simulink model "dx_hand_model_rai3"  (R2017b)
settings: Solver=ode3  StartTime=0.0  StopTime=inf  FixedStep=0.01  RelTol=1e-3  EnableMultiTasking=on
InitFcn:
  | cutFreq = 0.1; % T
  | sampleTime = 0.01;
  | filt = tf(1,[cutFreq 1]);
  | filt = c2d(filt,sampleTime);
  | 
  | cutFreq2 = 1;
  | filt2 = tf(1,[cutFreq2 1]);
  | filt2 = c2d(filt2,sampleTime);
  | 
  | update_param = 2;
  | 
  | ampliFactor = 1.60;
  | ampliFactorMiddle = 2.00;
  | ampliFactorDistal = 1;
  | 
  | % Set Hand Address
  | RightHandAddress = '10.24.4.91';
  | Verosim = '10.100.39.22'
  | LeftHandAddress = '10.24.4.90'
  | 
  | max_force = 12; % Newton
model workspace (MAT data in the model file):
  SL_ROS_VariableLengthArrays_MaxSizes : struct (value not decoded)
libraries: robotlib x134, simulink_extras x28, simulink x16, dspnetwork x5, etargetslib x4
(part 10 of 19)

== matlab function dx_hand_model_rai3/Middle Finger/Jacobian Calculation/Middle Jacobian ==
  data: pose input; sensor input; measurements input; JTcomp output single; q_next output; q_pr input; J22_old input; J22_ol output
function [JTcomp, q_next, J22_ol] = fcn( pose, sensor, measurements, q_pr, J22_old)
% La funzione e' stata modificata da Antonio in data 6/06/2018
%
%#codegen
%
lx = sensor(1);
qB = sensor(2);

qo1 =pose(1);
qo2 =pose(2);
qK = pose(3);
qD = pose(4);
qG = pose(5);
qN = pose(6);
c1 = pose(7);
c2 = pose(8);

s_slitta = 13.5;

%POSE ESTIMATION VALUE
xL_mag = measurements(3); % Posizione lungo l'asse x di L rispetto a K [RIMISURA]
offset = measurements(4); % Distanza tra il giunto K e l'appoggio del metacarpo [RIMISURA]
LIIp = measurements(1); % Semispessore del metacarpo e della falange (da tarare)
LIIp = LIIp + s_slitta;
LJJp = LIIp; % semispessore della falangina (da tarare, non per forza uguale a LIIp)
LLM = measurements(2); % Lunghezza della falange
LAB =  measurements(5);
LBC =  measurements(6);
LCD =  measurements(7);
LDE =  measurements(8);
LEF =  measurements(9);
LBH =  measurements(10); 
LGH =  measurements(11);
LGF =  measurements(12);
LEJ =  measurements(13);
LCI =  measurements(14);
LKB =  measurements(15);
LKNy = measurements(16); %% MISURA
LKNx = measurements(17); %% MISURA
lact = measurements(18); %Lunghezza dell'attuatore. [RIMISURA]

% LIIp = 7;
% LJJp = LIIp;
% LLM = 50;
% offset = 3;
% xL = 10;

% f1 = LLM;
% f5 = xL;
% LBH = 37; 
% LKB = 35;
% LKH = LKB + LBH;
% LCI = 16;
% LGH =  86;
LHG =  LGH;
% LDE = 40;
% LAB =  18;   
% LEF =  27;
% LGF =  46;
% LCD =  9;
% LBC =  43;
% oy  = 134.8;
% ox  = 15; 
% LEJ =  39;
% off_fing = LIIp;  
% lact = 117.77;
% LKN =  135.6320;
% LNO = lact;
% LDF = LDE + LEF;
% LBD = LBC + LCD;


stepsize = 0.01;

%%NEWEST (Jacobian_StiffnessRenderingOptimization_Sim.mdl)
q_dif = (sensor - q_pr) / stepsize;
q_dif1 = q_dif(1);
q_dif2 = q_dif(2);


J11 = -(cos(qo1)*(LKB*cos(qK)+LBC*cos(qB-qK)-LCI*sin(qB-qK))-sin(qo1)*(LKB*sin(qK)-LBC*sin(qB-qK)-LCI*cos(qB-qK)))*((LDE+LEF)*sin(qo2)*cos(qB-qD-qG)*(LKB*sin(qK)-LBC*sin(qB-qK)-LCI*cos(qB-qK))+(LDE+LEF)*sin(qN)^2*cos(qB-qD-qG)*(cos(qo1)*sin(qo1+qo2)*(LKB*sin(qK)-LBC*sin(qB-qK))-LCI*cos(qo1)*sin(qo1+qo2)*cos(qB-qK)-sin(qo2)*(LKB*sin(qK)-LBC*sin(qB-qK)-LCI*cos(qB-qK))-sin(qo1)*cos(qo1+qo2)*(LKB*sin(qK)-LBC*sin(qB-qK)-LCI*cos(qB-qK)))-cos(qo1)*((LDE+LEF)*cos(qB-qD-qG)*(cos(qo1+qo2)*(LCD*cos(qB-qK)+LCI*sin(qB-qK)+LDE*cos(qB-qD-qK)-LEJ*sin(qB-qD-qK))-sin(qo1+qo2)*(LCI*cos(qB-qK)-LCD*sin(qB-qK)-LDE*sin(qB-qD-qK)-LEJ*cos(qB-qD-qK)))+(sin(qo1+qo2)*(LDE*sin(qB-qD-qK)+LEJ*cos(qB-qD-qK))+cos(qo1+qo2)*(LDE*cos(qB-qD-qK)-LEJ*sin(qB-qD-qK)))*(cos(qG-qK)*(LBH*cos(qK)+LHG*sin(qK)-LBC*cos(qB-qK)-LCD*cos(qB-qK)-LDE*cos(qB-qD-qK)-LEF*cos(qB-qD-qK))+sin(qG-qK)*(LHG*cos(qK)-LBH*sin(qK)-LBC*sin(qB-qK)-LCD*sin(qB-qK)-LDE*sin(qB-qD-qK)-LEF*sin(qB-qD-qK)))))/(cos(qN)*(LKB*sin(qK)+LAB*sin(qB-qK)-tan(qN)*(LKB*cos(qK)-LAB*cos(qB-qK)))*((LDE+LEF)*sin(qo1)*sin(qo2)*cos(qB-qD-qG)*(LIIp*cos(qo1)-c1*sin(qo1))*(LKB*sin(qK)-LBC*sin(qB-qK)-LCI*cos(qB-qK))-cos(qo1)*((LIIp*sin(qo1)+c1*cos(qo1))*((LDE+LEF)*sin(qo2)*cos(qB-qD-qG)*(LKB*sin(qK)-LBC*sin(qB-qK)-LCI*cos(qB-qK))-cos(qo1)*((LDE+LEF)*cos(qB-qD-qG)*(cos(qo1+qo2)*(LCD*cos(qB-qK)+LCI*sin(qB-qK)+LDE*cos(qB-qD-qK)-LEJ*sin(qB-qD-qK))-sin(qo1+qo2)*(LCI*cos(qB-qK)-LCD*sin(qB-qK)-LDE*sin(qB-qD-qK)-LEJ*cos(qB-qD-qK)))+(sin(qo1+qo2)*(LDE*sin(qB-qD-qK)+LEJ*cos(qB-qD-qK))+cos(qo1+qo2)*(LDE*cos(qB-qD-qK)-LEJ*sin(qB-qD-qK)))*(cos(qG-qK)*(LBH*cos(qK)+LHG*sin(qK)-LBC*cos(qB-qK)-LCD*cos(qB-qK)-LDE*cos(qB-qD-qK)-LEF*cos(qB-qD-qK))+sin(qG-qK)*(LHG*cos(qK)-LBH*sin(qK)-LBC*sin(qB-qK)-LCD*sin(qB-qK)-LDE*sin(qB-qD-qK)-LEF*sin(qB-qD-qK)))))-sin(qo1)*(LIIp*cos(qo1)-c1*sin(qo1))*((LDE+LEF)*sin(qo1+qo2)*cos(qB-qD-qG)*(LCI*cos(qB-qK)-LCD*sin(qB-qK)-LDE*sin(qB-qD-qK)-LEJ*cos(qB-qD-qK))-sin(qo1+qo2)*(LDE*sin(qB-qD-qK)+LEJ*cos(qB-qD-qK))*(cos(qG-qK)*(LBH*cos(qK)+LHG*sin(qK)-LBC*cos(qB-qK)-LCD*cos(qB-qK)-LDE*cos(qB-qD-qK)-LEF*cos(qB-qD-qK))+sin(qG-qK)*(LHG*cos(qK)-LBH*sin(qK)-LBC*sin(qB-qK)-LCD*sin(qB-qK)-LDE*sin(qB-qD-qK)-LEF*sin(qB-qD-qK)))-cos(qo1+qo2)*((LDE+LEF)*cos(qG-qK)*cos(qB-qD-qK)*(LCD*cos(qB-qK)+LCI*sin(qB-qK)+LDE*cos(qB-qD-qK)-LEJ*sin(qB-qD-qK))+cos(qG-qK)*(LDE*cos(qB-qD-qK)-LEJ*sin(qB-qD-qK))*(LBH*cos(qK)+LHG*sin(qK)-LBC*cos(qB-qK)-LCD*cos(qB-qK)-LDE*cos(qB-qD-qK)-LEF*cos(qB-qD-qK))+sin(qG-qK)*((LDE+LEF)*sin(qB-qD-qK)*(LCD*cos(qB-qK)+LCI*sin(qB-qK)+LDE*cos(qB-qD-qK)-LEJ*sin(qB-qD-qK))+(LDE*cos(qB-qD-qK)-LEJ*sin(qB-qD-qK))*(LHG*cos(qK)-LBH*sin(qK)-LBC*sin(qB-qK)-LCD*sin(qB-qK)-LDE*sin(qB-qD-qK)-LEF*sin(qB-qD-qK))))))));
J12 = cos(qo1)*((LDE+LEF)*sin(qo1+qo2)*cos(qB-qD-qG)*(LCI*cos(qB-qK)-LCD*sin(qB-qK)-LDE*sin(qB-qD-qK)-LEJ*cos(qB-qD-qK))*(cos(qo1)*(LKB*cos(qK)+LBC*cos(qB-qK)-LCI*sin(qB-qK))-sin(qo1)*(LKB*sin(qK)-LBC*sin(qB-qK)-LCI*cos(qB-qK)))+sin(qG-qK)*(LBC*sin(qB-qK)+LCD*sin(qB-qK)+LDE*sin(qB-qD-qK)+LEF*sin(qB-qD-qK))*(sin(qo1+qo2)*(LDE*sin(qB-qD-qK)+LEJ*cos(qB-qD-qK))+cos(qo1+qo2)*(LDE*cos(qB-qD-qK)-LEJ*sin(qB-qD-qK)))*(cos(qo1)*(LKB*cos(qK)+LBC*cos(qB-qK)-LCI*sin(qB-qK))-sin(qo1)*(LKB*sin(qK)-LBC*sin(qB-qK)-LCI*cos(qB-qK)))+cos(qG-qK)*(LBC*cos(qB-qK)+LCD*cos(qB-qK)+LDE*cos(qB-qD-qK)+LEF*cos(qB-qD-qK))*(sin(qo1+qo2)*(LDE*sin(qB-qD-qK)+LEJ*cos(qB-qD-qK))+cos(qo1+qo2)*(LDE*cos(qB-qD-qK)-LEJ*sin(qB-qD-qK)))*(cos(qo1)*(LKB*cos(qK)+LBC*cos(qB-qK)-LCI*sin(qB-qK))-sin(qo1)*(LKB*sin(qK)-LBC*sin(qB-qK)-LCI*cos(qB-qK)))-(LDE+LEF)*cos(qo1+qo2)*cos(qB-qD-qG)*(LCD*cos(qB-qK)+LCI*sin(qB-qK)+LDE*cos(qB-qD-qK)-LEJ*sin(qB-qD-qK))*(cos(qo1)*(LKB*cos(qK)+LBC*cos(qB-qK)-LCI*sin(qB-qK))-sin(qo1)*(LKB*sin(qK)-LBC*sin(qB-qK)-LCI*cos(qB-qK)))-(LBC*cos(qB-qK)-LCI*sin(qB-qK))*((LDE+LEF)*sin(qo2)*cos(qB-qD-qG)*(LKB*sin(qK)-LBC*sin(qB-qK)-LCI*cos(qB-qK))-cos(qo1)*((LDE+LEF)*cos(qB-qD-qG)*(cos(qo1+qo2)*(LCD*cos(qB-qK)+LCI*sin(qB-qK)+LDE*cos(qB-qD-qK)-LEJ*sin(qB-qD-qK))-sin(qo1+qo2)*(LCI*cos(qB-qK)-LCD*sin(qB-qK)-LDE*sin(qB-qD-qK)-LEJ*cos(qB-qD-qK)))+(sin(qo1+qo2)*(LDE*sin(qB-qD-qK)+LEJ*cos(qB-qD-qK))+cos(qo1+qo2)*(LDE*cos(qB-qD-qK)-LEJ*sin(qB-qD-qK)))*(cos(qG-qK)*(LBH*cos(qK)+LHG*sin(qK)-LBC*cos(qB-qK)-LCD*cos(qB-qK)-LDE*cos(qB-qD-qK)-LEF*cos(qB-qD-qK))+sin(qG-qK)*(LHG*cos(qK)-LBH*sin(qK)-LBC*sin(qB-qK)-LCD*sin(qB-qK)-LDE*sin(qB-qD-qK)-LEF*sin(qB-qD-qK)))))-(LBC*sin(qB-qK)+LCI*cos(qB-qK))*((LDE+LEF)*sin(qo2)*cos(qB-qD-qG)*(LKB*cos(qK)+LBC*cos(qB-qK)-LCI*sin(qB-qK))+sin(qo1)*((LDE+LEF)*sin(qo1+qo2)*cos(qB-qD-qG)*(LCI*cos(qB-qK)-LCD*sin(qB-qK)-LDE*sin(qB-qD-qK)-LEJ*cos(qB-qD-qK))-sin(qo1+qo2)*(LDE*sin(qB-qD-qK)+LEJ*cos(qB-qD-qK))*(cos(qG-qK)*(LBH*cos(qK)+LHG*sin(qK)-LBC*cos(qB-qK)-LCD*cos(qB-qK)-LDE*cos(qB-qD-qK)-LEF*cos(qB-qD-qK))+sin(qG-qK)*(LHG*cos(qK)-LBH*sin(qK)-LBC*sin(qB-qK)-LCD*sin(qB-qK)-LDE*sin(qB-qD-qK)-LEF*sin(qB-qD-qK)))-cos(qo1+qo2)*((LDE+LEF)*cos(qG-qK)*cos(qB-qD-qK)*(LCD*cos(qB-qK)+LCI*sin(qB-qK)+LDE*cos(qB-qD-qK)-LEJ*sin(qB-qD-qK))+cos(qG-qK)*(LDE*cos(qB-qD-qK)-LEJ*sin(qB-qD-qK))*(LBH*cos(qK)+LHG*sin(qK)-LBC*cos(qB-qK)-LCD*cos(qB-qK)-LDE*cos(qB-qD-qK)-LEF*cos(qB-qD-qK))+sin(qG-qK)*((LDE+LEF)*sin(qB-qD-qK)*(LCD*cos(qB-qK)+LCI*sin(qB-qK)+LDE*cos(qB-qD-qK)-LEJ*sin(qB-qD-qK))+(LDE*cos(qB-qD-qK)-LEJ*sin(qB-qD-qK))*(LHG*cos(qK)-LBH*sin(qK)-LBC*sin(qB-qK)-LCD*sin(qB-qK)-LDE*sin(qB-qD-qK)-LEF*sin(qB-qD-qK)))))))/((LDE+LEF)*sin(qo1)*sin(qo2)*cos(qB-qD-qG)*(LIIp*cos(qo1)-c1*sin(qo1))*(LKB*sin(qK)-LBC*sin(qB-qK)-LCI*cos(qB-qK))-cos(qo1)*((LIIp*sin(qo1)+c1*cos(qo1))*((LDE+LEF)*sin(qo2)*cos(qB-qD-qG)*(LKB*sin(qK)-LBC*sin(qB-qK)-LCI*cos(qB-qK))-cos(qo1)*((LDE+LEF)*cos(qB-qD-qG)*(cos(qo1+qo2)*(LCD*cos(qB-qK)+LCI*sin(qB-qK)+LDE*cos(qB-qD-qK)-LEJ*sin(qB-qD-qK))-sin(qo1+qo2)*(LCI*cos(qB-qK)-LCD*sin(qB-qK)-LDE*sin(qB-qD-qK)-LEJ*cos(qB-qD-qK)))+(sin(qo1+qo2)*(LDE*sin(qB-qD-qK)+LEJ*cos(qB-qD-qK))+cos(qo1+qo2)*(LDE*cos(qB-qD-qK)-LEJ*sin(qB-qD-qK)))*(cos(qG-qK)*(LBH*cos(qK)+LHG*sin(qK)-LBC*cos(qB-qK)-LCD*cos(qB-qK)-LDE*cos(qB-qD-qK)-LEF*cos(qB-qD-qK))+sin(qG-qK)*(LHG*cos(qK)-LBH*sin(qK)-LBC*sin(qB-qK)-LCD*sin(qB-qK)-LDE*sin(qB-qD-qK)-LEF*sin(qB-qD-qK)))))-sin(qo1)*(LIIp*cos(qo1)-c1*sin(qo1))*((LDE+LEF)*sin(qo1+qo2)*cos(qB-qD-qG)*(LCI*cos(qB-qK)-LCD*sin(qB-qK)-LDE*sin(qB-qD-qK)-LEJ*cos(qB-qD-qK))-sin(qo1+qo2)*(LDE*sin(qB-qD-qK)+LEJ*cos(qB-qD-qK))*(cos(qG-qK)*(LBH*cos(qK)+LHG*sin(qK)-LBC*cos(qB-qK)-LCD*cos(qB-qK)-LDE*cos(qB-qD-qK)-LEF*cos(qB-qD-qK))+sin(qG-qK)*(LHG*cos(qK)-LBH*sin(qK)-LBC*sin(qB-qK)-LCD*sin(qB-qK)-LDE*sin(qB-qD-qK)-LEF*sin(qB-qD-qK)))-cos(qo1+qo2)*((LDE+LEF)*cos(qG-qK)*cos(qB-qD-qK)*(LCD*cos(qB-qK)+LCI*sin(qB-qK)+LDE*cos(qB-qD-qK)-LEJ*sin(qB-qD-qK))+cos(qG-qK)*(LDE*cos(qB-qD-qK)-LEJ*sin(qB-qD-qK))*(LBH*cos(qK)+LHG*sin(qK)-LBC*cos(qB-qK)-LCD*cos(qB-qK)-LDE*cos(qB-qD-qK)-LEF*cos(qB-qD-qK))+sin(qG-qK)*((LDE+LEF)*sin(qB-qD-qK)*(LCD*cos(qB-qK)+LCI*sin(qB-qK)+LDE*cos(qB-qD-qK)-LEJ*sin(qB-qD-qK))+(LDE*cos(qB-qD-qK)-LEJ*sin(qB-qD-qK))*(LHG*cos(qK)-LBH*sin(qK)-LBC*sin(qB-qK)-LCD*sin(qB-qK)-LDE*sin(qB-qD-qK)-LEF*sin(qB-qD-qK))))))) - (cos(qo1)*(LKB*cos(qK)+LBC*cos(qB-qK)-LCI*sin(qB-qK))-sin(qo1)*(LKB*sin(qK)-LBC*sin(qB-qK)-LCI*cos(qB-qK)))*((LDE+LEF)*cos(qo1)*sin(qo1+qo2)*cos(qB-qD-qG)*(LKB*sin(qK)+LAB*sin(qB-qK)-tan(qN)*(LKB*cos(qK)-LAB*cos(qB-qK)))*(LCI*cos(qB-qK)-LCD*sin(qB-qK)-LDE*sin(qB-qD-qK)-LEJ*cos(qB-qD-qK))+cos(qo1)*sin(qG-qK)*(LKB*sin(qK)+LAB*sin(qB-qK)-tan(qN)*(LKB*cos(qK)-LAB*cos(qB-qK)))*(LBC*sin(qB-qK)+LCD*sin(qB-qK)+LDE*sin(qB-qD-qK)+LEF*sin(qB-qD-qK))*(sin(qo1+qo2)*(LDE*sin(qB-qD-qK)+LEJ*cos(qB-qD-qK))+cos(qo1+qo2)*(LDE*cos(qB-qD-qK)-LEJ*sin(qB-qD-qK)))+cos(qo1)*cos(qG-qK)*(LKB*sin(qK)+LAB*sin(qB-qK)-tan(qN)*(LKB*cos(qK)-LAB*cos(qB-qK)))*(LBC*cos(qB-qK)+LCD*cos(qB-qK)+LDE*cos(qB-qD-qK)+LEF*cos(qB-qD-qK))*(sin(qo1+qo2)*(LDE*sin(qB-qD-qK)+LEJ*cos(qB-qD-qK))+cos(qo1+qo2)*(LDE*cos(qB-qD-qK)-LEJ*sin(qB-qD-qK)))-(LDE+LEF)*sin(qo2)*cos(qB-qD-qG)*(LBC*sin(qB-qK)+LCI*cos(qB-qK))*(LKB*sin(qK)+LAB*sin(qB-qK)-tan(qN)*(LKB*cos(qK)-LAB*cos(qB-qK)))-(LDE+LEF)*cos(qo1)*cos(qo1+qo2)*cos(qB-qD-qG)*(LKB*sin(qK)+LAB*sin(qB-qK)-tan(qN)*(LKB*cos(qK)-LAB*cos(qB-qK)))*(LCD*cos(qB-qK)+LCI*sin(qB-qK)+LDE*cos(qB-qD-qK)-LEJ*sin(qB-qD-qK))-LAB*sin(qB-qK)*((LDE+LEF)*sin(qo2)*cos(qB-qD-qG)*(LKB*sin(qK)-LBC*sin(qB-qK)-LCI*cos(qB-qK))-cos(qo1)*((LDE+LEF)*cos(qB-qD-qG)*(cos(qo1+qo2)*(LCD*cos(qB-qK)+LCI*sin(qB-qK)+LDE*cos(qB-qD-qK)-LEJ*sin(qB-qD-qK))-sin(qo1+qo2)*(LCI*cos(qB-qK)-LCD*sin(qB-qK)-LDE*sin(qB-qD-qK)-LEJ*cos(qB-qD-qK)))+(sin(qo1+qo2)*(LDE*sin(qB-qD-qK)+LEJ*cos(qB-qD-qK))+cos(qo1+qo2)*(LDE*cos(qB-qD-qK)-LEJ*sin(qB-qD-qK)))*(cos(qG-qK)*(LBH*cos(qK)+LHG*sin(qK)-LBC*cos(qB-qK)-LCD*cos(qB-qK)-LDE*cos(qB-qD-qK)-LEF*cos(qB-qD-qK))+sin(qG-qK)*(LHG*cos(qK)-LBH*sin(qK)-LBC*sin(qB-qK)-LCD*sin(qB-qK)-LDE*sin(qB-qD-qK)-LEF*sin(qB-qD-qK)))))-LAB*tan(qN)*cos(qB-qK)*((LDE+LEF)*cos(qo1)*sin(qo1+qo2)*cos(qB-qD-qG)*(LKB*sin(qK)-LBC*sin(qB-qK)-LCD*sin(qB-qK)-LDE*sin(qB-qD-qK)-LEJ*cos(qB-qD-qK))-(LDE+LEF)*sin(qo1)*cos(qo1+qo2)*cos(qB-qD-qG)*(LKB*sin(qK)-LBC*sin(qB-qK)-LCI*cos(qB-qK))-cos(qo1)*sin(qo1+qo2)*(LDE*sin(qB-qD-qK)+LEJ*cos(qB-qD-qK))*(cos(qG-qK)*(LBH*cos(qK)+LHG*sin(qK)-LBC*cos(qB-qK)-LCD*cos(qB-qK)-LDE*cos(qB-qD-qK)-LEF*cos(qB-qD-qK))+sin(qG-qK)*(LHG*cos(qK)-LBH*sin(qK)-LBC*sin(qB-qK)-LCD*sin(qB-qK)-LDE*sin(qB-qD-qK)-LEF*sin(qB-qD-qK)))-cos(qo1)*cos(qo1+qo2)*((LDE+LEF)*cos(qG-qK)*cos(qB-qD-qK)*(LCD*cos(qB-qK)+LCI*sin(qB-qK)+LDE*cos(qB-qD-qK)-LEJ*sin(qB-qD-qK))+cos(qG-qK)*(LDE*cos(qB-qD-qK)-LEJ*sin(qB-qD-qK))*(LBH*cos(qK)+LHG*sin(qK)-LBC*cos(qB-qK)-LCD*cos(qB-qK)-LDE*cos(qB-qD-qK)-LEF*cos(qB-qD-qK))+sin(qG-qK)*((LDE+LEF)*sin(qB-qD-qK)*(LCD*cos(qB-qK)+LCI*sin(qB-qK)+LDE*cos(qB-qD-qK)-LEJ*sin(qB-qD-qK))+(LDE*cos(qB-qD-qK)-LEJ*sin(qB-qD-qK))*(LHG*cos(qK)-LBH*sin(qK)-LBC*sin(qB-qK)-LCD*sin(qB-qK)-LDE*sin(qB-qD-qK)-LEF*sin(qB-qD-qK))))))/((LKB*sin(qK)+LAB*sin(qB-qK)-tan(qN)*(LKB*cos(qK)-LAB*cos(qB-qK)))*((LDE+LEF)*sin(qo1)*sin(qo2)*cos(qB-qD-qG)*(LIIp*cos(qo1)-c1*sin(qo1))*(LKB*sin(qK)-LBC*sin(qB-qK)-LCI*cos(qB-qK))-cos(qo1)*((LIIp*sin(qo1)+c1*cos(qo1))*((LDE+LEF)*sin(qo2)*cos(qB-qD-qG)*(LKB*sin(qK)-LBC*sin(qB-qK)-LCI*cos(qB-qK))-cos(qo1)*((LDE+LEF)*cos(qB-qD-qG)*(cos(qo1+qo2)*(LCD*cos(qB-qK)+LCI*sin(qB-qK)+LDE*cos(qB-qD-qK)-LEJ*sin(qB-qD-qK))-sin(qo1+qo2)*(LCI*cos(qB-qK)-LCD*sin(qB-qK)-LDE*sin(qB-qD-qK)-LEJ*cos(qB-qD-qK)))+(sin(qo1+qo2)*(LDE*sin(qB-qD-qK)+LEJ*cos(qB-qD-qK))+cos(qo1+qo2)*(LDE*cos(qB-qD-qK)-LEJ*sin(qB-qD-qK)))*(cos(qG-qK)*(LBH*cos(qK)+LHG*sin(qK)-LBC*cos(qB-qK)-LCD*cos(qB-qK)-LDE*cos(qB-qD-qK)-LEF*cos(qB-qD-qK))+sin(qG-qK)*(LHG*cos(qK)-LBH*sin(qK)-LBC*sin(qB-qK)-LCD*sin(qB-qK)-LDE*sin(qB-qD-qK)-LEF*sin(qB-qD-qK)))))-sin(qo1)*(LIIp*cos(qo1)-c1*sin(qo1))*((LDE+LEF)*sin(qo1+qo2)*cos(qB-qD-qG)*(LCI*cos(qB-qK)-LCD*sin(qB-qK)-LDE*sin(qB-qD-qK)-LEJ*cos(qB-qD-qK))-sin(qo1+qo2)*(LDE*sin(qB-qD-qK)+LEJ*cos(qB-qD-qK))*(cos(qG-qK)*(LBH*cos(qK)+LHG*sin(qK)-LBC*cos(qB-qK)-LCD*cos(qB-qK)-LDE*cos(qB-qD-qK)-LEF*cos(qB-qD-qK))+sin(qG-qK)*(LHG*cos(qK)-LBH*sin(qK)-LBC*sin(qB-qK)-LCD*sin(qB-qK)-LDE*sin(qB-qD-qK)-LEF*sin(qB-qD-qK)))-cos(qo1+qo2)*((LDE+LEF)*cos(qG-qK)*cos(qB-qD-qK)*(LCD*cos(qB-qK)+LCI*sin(qB-qK)+LDE*cos(qB-qD-qK)-LEJ*sin(qB-qD-qK))+cos(qG-qK)*(LDE*cos(qB-qD-qK)-LEJ*sin(qB-qD-qK))*(LBH*cos(qK)+LHG*sin(qK)-LBC*cos(qB-qK)-LCD*cos(qB-qK)-LDE*cos(qB-qD-qK)-LEF*cos(qB-qD-qK))+sin(qG-qK)*((LDE+LEF)*sin(qB-qD-qK)*(LCD*cos(qB-qK)+LCI*sin(qB-qK)+LDE*cos(qB-qD-qK)-LEJ*sin(qB-qD-qK))+(LDE*cos(qB-qD-qK)-LEJ*sin(qB-qD-qK))*(LHG*cos(qK)-LBH*sin(qK)-LBC*sin(qB-qK)-LCD*sin(qB-qK)-LDE*sin(qB-qD-qK)-LEF*sin(qB-qD-qK))))))));
J21 = -(((LDE+LEF)*sin(qo2)*cos(qB-qD-qG)*(LKB*sin(qK)-LBC*sin(qB-qK)-LCI*cos(qB-qK))-cos(qo1)*((LDE+LEF)*cos(qB-qD-qG)*(cos(qo1+qo2)*(LCD*cos(qB-qK)+LCI*sin(qB-qK)+LDE*cos(qB-qD-qK)-LEJ*sin(qB-qD-qK))-sin(qo1+qo2)*(LCI*cos(qB-qK)-LCD*sin(qB-qK)-LDE*sin(qB-qD-qK)-LEJ*cos(qB-qD-qK)))+(sin(qo1+qo2)*(LDE*sin(qB-qD-qK)+LEJ*cos(qB-qD-qK))+cos(qo1+qo2)*(LDE*cos(qB-qD-qK)-LEJ*sin(qB-qD-qK)))*(cos(qG-qK)*(LBH*cos(qK)+LHG*sin(qK)-LBC*cos(qB-qK)-LCD*cos(qB-qK)-LDE*cos(qB-qD-qK)-LEF*cos(qB-qD-qK))+sin(qG-qK)*(LHG*cos(qK)-LBH*sin(qK)-LBC*sin(qB-qK)-LCD*sin(qB-qK)-LDE*sin(qB-qD-qK)-LEF*sin(qB-qD-qK)))))^2*(cos(qN)+sin(qN)^2*((LDE+LEF)*cos(qo1)*sin(qo1+qo2)*cos(qB-qD-qG)*(LKB*sin(qK)-LBC*sin(qB-qK)-LCD*sin(qB-qK)-LDE*sin(qB-qD-qK)-LEJ*cos(qB-qD-qK))-(LDE+LEF)*sin(qo1)*cos(qo1+qo2)*cos(qB-qD-qG)*(LKB*sin(qK)-LBC*sin(qB-qK)-LCI*cos(qB-qK))-cos(qo1)*sin(qo1+qo2)*(LDE*sin(qB-qD-qK)+LEJ*cos(qB-qD-qK))*(cos(qG-qK)*(LBH*cos(qK)+LHG*sin(qK)-LBC*cos(qB-qK)-LCD*cos(qB-qK)-LDE*cos(qB-qD-qK)-LEF*cos(qB-qD-qK))+sin(qG-qK)*(LHG*cos(qK)-LBH*sin(qK)-LBC*sin(qB-qK)-LCD*sin(qB-qK)-LDE*sin(qB-qD-qK)-LEF*sin(qB-qD-qK)))-cos(qo1)*cos(qo1+qo2)*((LDE+LEF)*cos(qG-qK)*cos(qB-qD-qK)*(LCD*cos(qB-qK)+LCI*sin(qB-qK)+LDE*cos(qB-qD-qK)-LEJ*sin(qB-qD-qK))+cos(qG-qK)*(LDE*cos(qB-qD-qK)-LEJ*sin(qB-qD-qK))*(LBH*cos(qK)+LHG*sin(qK)-LBC*cos(qB-qK)-LCD*cos(qB-qK)-LDE*cos(qB-qD-qK)-LEF*cos(qB-qD-qK))+sin(qG-qK)*((LDE+LEF)*sin(qB-qD-qK)*(LCD*cos(qB-qK)+LCI*sin(qB-qK)+LDE*cos(qB-qD-qK)-LEJ*sin(qB-qD-qK))+(LDE*cos(qB-qD-qK)-LEJ*sin(qB-qD-qK))*(LHG*cos(qK)-LBH*sin(qK)-LBC*sin(qB-qK)-LCD*sin(qB-qK)-LDE*sin(qB-qD-qK)-LEF*sin(qB-qD-qK)))))/(cos(qN)*((LDE+LEF)*sin(qo2)*cos(qB-qD-qG)*(LKB*sin(qK)-LBC*sin(qB-qK)-LCI*cos(qB-qK))-cos(qo1)*((LDE+LEF)*cos(qB-qD-qG)*(cos(qo1+qo2)*(LCD*cos(qB-qK)+LCI*sin(qB-qK)+LDE*cos(qB-qD-qK)-LEJ*sin(qB-qD-qK))-sin(qo1+qo2)*(LCI*cos(qB-qK)-LCD*sin(qB-qK)-LDE*sin(qB-qD-qK)-LEJ*cos(qB-qD-qK)))+(sin(qo1+qo2)*(LDE*sin(qB-qD-qK)+LEJ*cos(qB-qD-qK))+cos(qo1+qo2)*(LDE*cos(qB-qD-qK)-LEJ*sin(qB-qD-qK)))*(cos(qG-qK)*(LBH*cos(qK)+LHG*sin(qK)-LBC*cos(qB-qK)-LCD*cos(qB-qK)-LDE*cos(qB-qD-qK)-LEF*cos(qB-qD-qK))+sin(qG-qK)*(LHG*cos(qK)-LBH*sin(qK)-LBC*sin(qB-qK)-LCD*sin(qB-qK)-LDE*sin(qB-qD-qK)-LEF*sin(qB-qD-qK)))))))*(LIIp*sin(qo1)+c1*cos(qo1)+((LDE+LEF)*c2*cos(qB-qD-qG)*(cos(qo1)*(LKB*cos(qK)+LBC*cos(qB-qK)-LCI*sin(qB-qK))-sin(qo1)*(LKB*sin(qK)-LBC*sin(qB-qK)-LCI*cos(qB-qK)))+(LDE+LEF)*sin(qo1+qo2)*cos(qB-qD-qG)*(LIIp*cos(qo1)+sin(qo1)*(LLM-c1))*(cos(qo1)*(LKB*cos(qK)+LBC*cos(qB-qK)-LCI*sin(qB-qK))-sin(qo1)*(LKB*sin(qK)-LBC*sin(qB-qK)-LCI*cos(qB-qK)))-(LDE+LEF)*cos(qo1+qo2)*cos(qB-qD-qG)*(LIIp*sin(qo1)-cos(qo1)*(LLM-c1))*(cos(qo1)*(LKB*cos(qK)+LBC*cos(qB-qK)-LCI*sin(qB-qK))-sin(qo1)*(LKB*sin(qK)-LBC*sin(qB-qK)-LCI*cos(qB-qK)))-(LIIp*cos(qo1)-c1*sin(qo1))*((LDE+LEF)*sin(qo2)*cos(qB-qD-qG)*(LKB*cos(qK)+LBC*cos(qB-qK)-LCI*sin(qB-qK))+sin(qo1)*((LDE+LEF)*sin(qo1+qo2)*cos(qB-qD-qG)*(LCI*cos(qB-qK)-LCD*sin(qB-qK)-LDE*sin(qB-qD-qK)-LEJ*cos(qB-qD-qK))-sin(qo1+qo2)*(LDE*sin(qB-qD-qK)+LEJ*cos(qB-qD-qK))*(cos(qG-qK)*(LBH*cos(qK)+LHG*sin(qK)-LBC*cos(qB-qK)-LCD*cos(qB-qK)-LDE*cos(qB-qD-qK)-LEF*cos(qB-qD-qK))+sin(qG-qK)*(LHG*cos(qK)-LBH*sin(qK)-LBC*sin(qB-qK)-LCD*sin(qB-qK)-LDE*sin(qB-qD-qK)-LEF*sin(qB-qD-qK)))-cos(qo1+qo2)*((LDE+LEF)*cos(qG-qK)*cos(qB-qD-qK)*(LCD*cos(qB-qK)+LCI*sin(qB-qK)+LDE*cos(qB-qD-qK)-LEJ*sin(qB-qD-qK))+cos(qG-qK)*(LDE*cos(qB-qD-qK)-LEJ*sin(qB-qD-qK))*(LBH*cos(qK)+LHG*sin(qK)-LBC*cos(qB-qK)-LCD*cos(qB-qK)-LDE*cos(qB-qD-qK)-LEF*cos(qB-qD-qK))+sin(qG-qK)*((LDE+LEF)*sin(qB-qD-qK)*(LCD*cos(qB-qK)+LCI*sin(qB-qK)+LDE*cos(qB-qD-qK)-LEJ*sin(qB-qD-qK))+(LDE*cos(qB-qD-qK)-LEJ*sin(qB-qD-qK))*(LHG*cos(qK)-LBH*sin(qK)-LBC*sin(qB-qK)-LCD*sin(qB-qK)-LDE*sin(qB-qD-qK)-LEF*sin(qB-qD-qK)))))))/((LDE+LEF)*sin(qo2)*cos(qB-qD-qG)*(LKB*sin(qK)-LBC*sin(qB-qK)-LCI*cos(qB-qK))-cos(qo1)*((LDE+LEF)*cos(qB-qD-qG)*(cos(qo1+qo2)*(LCD*cos(qB-qK)+LCI*sin(qB-qK)+LDE*cos(qB-qD-qK)-LEJ*sin(qB-qD-qK))-sin(qo1+qo2)*(LCI*cos(qB-qK)-LCD*sin(qB-qK)-LDE*sin(qB-qD-qK)-LEJ*cos(qB-qD-qK)))+(sin(qo1+qo2)*(LDE*sin(qB-qD-qK)+LEJ*cos(qB-qD-qK))+cos(qo1+qo2)*(LDE*cos(qB-qD-qK)-LEJ*sin(qB-qD-qK)))*(cos(qG-qK)*(LBH*cos(qK)+LHG*sin(qK)-LBC*cos(qB-qK)-LCD*cos(qB-qK)-LDE*cos(qB-qD-qK)-LEF*cos(qB-qD-qK))+sin(qG-qK)*(LHG*cos(qK)-LBH*sin(qK)-LBC*sin(qB-qK)-LCD*sin(qB-qK)-LDE*sin(qB-qD-qK)-LEF*sin(qB-qD-qK))))))/((LDE+LEF)*c2*cos(qB-qD-qG)*(LKB*sin(qK)+LAB*sin(qB-qK)-tan(qN)*(LKB*cos(qK)-LAB*cos(qB-qK)))*((LDE+LEF)*sin(qo1)*sin(qo2)*cos(qB-qD-qG)*(LIIp*cos(qo1)-c1*sin(qo1))*(LKB*sin(qK)-LBC*sin(qB-qK)-LCI*cos(qB-qK))-cos(qo1)*((LIIp*sin(qo1)+c1*cos(qo1))*((LDE+LEF)*sin(qo2)*cos(qB-qD-qG)*(LKB*sin(qK)-LBC*sin(qB-qK)-LCI*cos(qB-qK))-cos(qo1)*((LDE+LEF)*cos(qB-qD-qG)*(cos(qo1+qo2)*(LCD*cos(qB-qK)+LCI*sin(qB-qK)+LDE*cos(qB-qD-qK)-LEJ*sin(qB-qD-qK))-sin(qo1+qo2)*(LCI*cos(qB-qK)-LCD*sin(qB-qK)-LDE*sin(qB-qD-qK)-LEJ*cos(qB-qD-qK)))+(sin(qo1+qo2)*(LDE*sin(qB-qD-qK)+LEJ*cos(qB-qD-qK))+cos(qo1+qo2)*(LDE*cos(qB-qD-qK)-LEJ*sin(qB-qD-qK)))*(cos(qG-qK)*(LBH*cos(qK)+LHG*sin(qK)-LBC*cos(qB-qK)-LCD*cos(qB-qK)-LDE*cos(qB-qD-qK)-LEF*cos(qB-qD-qK))+sin(qG-qK)*(LHG*cos(qK)-LBH*sin(qK)-LBC*sin(qB-qK)-LCD*sin(qB-qK)-LDE*sin(qB-qD-qK)-LEF*sin(qB-qD-qK)))))-sin(qo1)*(LIIp*cos(qo1)-c1*sin(qo1))*((LDE+LEF)*sin(qo1+qo2)*cos(qB-qD-qG)*(LCI*cos(qB-qK)-LCD*sin(qB-qK)-LDE*sin(qB-qD-qK)-LEJ*cos(qB-qD-qK))-sin(qo1+qo2)*(LDE*sin(qB-qD-qK)+LEJ*cos(qB-qD-qK))*(cos(qG-qK)*(LBH*cos(qK)+LHG*sin(qK)-LBC*cos(qB-qK)-LCD*cos(qB-qK)-LDE*cos(qB-qD-qK)-LEF*cos(qB-qD-qK))+sin(qG-qK)*(LHG*cos(qK)-LBH*sin(qK)-LBC*sin(qB-qK)-LCD*sin(qB-qK)-LDE*sin(qB-qD-qK)-LEF*sin(qB-qD-qK)))-cos(qo1+qo2)*((LDE+LEF)*cos(qG-qK)*cos(qB-qD-qK)*(LCD*cos(qB-qK)+LCI*sin(qB-qK)+LDE*cos(qB-qD-qK)-LEJ*sin(qB-qD-qK))+cos(qG-qK)*(LDE*cos(qB-qD-qK)-LEJ*sin(qB-qD-qK))*(LBH*cos(qK)+LHG*sin(qK)-LBC*cos(qB-qK)-LCD*cos(qB-qK)-LDE*cos(qB-qD-qK)-LEF*cos(qB-qD-qK))+sin(qG-qK)*((LDE+LEF)*sin(qB-qD-qK)*(LCD*cos(qB-qK)+LCI*sin(qB-qK)+LDE*cos(qB-qD-qK)-LEJ*sin(qB-qD-qK))+(LDE*cos(qB-qD-qK)-LEJ*sin(qB-qD-qK))*(LHG*cos(qK)-LBH*sin(qK)-LBC*sin(qB-qK)-LCD*sin(qB-qK)-LDE*sin(qB-qD-qK)-LEF*sin(qB-qD-qK)))))))));
J22_c = (-(c2*cos(qo1)+cos(qo1)*sin(qo1+qo2)*(LIIp*cos(qo1)+sin(qo1)*(LLM-c1))-sin(qo2)*(LIIp*cos(qo1)-c1*sin(qo1))-cos(qo1)*cos(qo1+qo2)*(LIIp*sin(qo1)-cos(qo1)*(LLM-c1)))*((LDE+LEF)*sin(qo1+qo2)*cos(qB-qD-qG)*(LCI*cos(qB-qK)-LCD*sin(qB-qK)-LDE*sin(qB-qD-qK)-LEJ*cos(qB-qD-qK))*(cos(qo1)*(LKB*cos(qK)+LBC*cos(qB-qK)-LCI*sin(qB-qK))-sin(qo1)*(LKB*sin(qK)-LBC*sin(qB-qK)-LCI*cos(qB-qK)))+sin(qG-qK)*(LBC*sin(qB-qK)+LCD*sin(qB-qK)+LDE*sin(qB-qD-qK)+LEF*sin(qB-qD-qK))*(sin(qo1+qo2)*(LDE*sin(qB-qD-qK)+LEJ*cos(qB-qD-qK))+cos(qo1+qo2)*(LDE*cos(qB-qD-qK)-LEJ*sin(qB-qD-qK)))*(cos(qo1)*(LKB*cos(qK)+LBC*cos(qB-qK)-LCI*sin(qB-qK))-sin(qo1)*(LKB*sin(qK)-LBC*sin(qB-qK)-LCI*cos(qB-qK)))+cos(qG-qK)*(LBC*cos(qB-qK)+LCD*cos(qB-qK)+LDE*cos(qB-qD-qK)+LEF*cos(qB-qD-qK))*(sin(qo1+qo2)*(LDE*sin(qB-qD-qK)+LEJ*cos(qB-qD-qK))+cos(qo1+qo2)*(LDE*cos(qB-qD-qK)-LEJ*sin(qB-qD-qK)))*(cos(qo1)*(LKB*cos(qK)+LBC*cos(qB-qK)-LCI*sin(qB-qK))-sin(qo1)*(LKB*sin(qK)-LBC*sin(qB-qK)-LCI*cos(qB-qK)))-(LDE+LEF)*cos(qo1+qo2)*cos(qB-qD-qG)*(LCD*cos(qB-qK)+LCI*sin(qB-qK)+LDE*cos(qB-qD-qK)-LEJ*sin(qB-qD-qK))*(cos(qo1)*(LKB*cos(qK)+LBC*cos(qB-qK)-LCI*sin(qB-qK))-sin(qo1)*(LKB*sin(qK)-LBC*sin(qB-qK)-LCI*cos(qB-qK)))-(LBC*cos(qB-qK)-LCI*sin(qB-qK))*((LDE+LEF)*sin(qo2)*cos(qB-qD-qG)*(LKB*sin(qK)-LBC*sin(qB-qK)-LCI*cos(qB-qK))-cos(qo1)*((LDE+LEF)*cos(qB-qD-qG)*(cos(qo1+qo2)*(LCD*cos(qB-qK)+LCI*sin(qB-qK)+LDE*cos(qB-qD-qK)-LEJ*sin(qB-qD-qK))-sin(qo1+qo2)*(LCI*cos(qB-qK)-LCD*sin(qB-qK)-LDE*sin(qB-qD-qK)-LEJ*cos(qB-qD-qK)))+(sin(qo1+qo2)*(LDE*sin(qB-qD-qK)+LEJ*cos(qB-qD-qK))+cos(qo1+qo2)*(LDE*cos(qB-qD-qK)-LEJ*sin(qB-qD-qK)))*(cos(qG-qK)*(LBH*cos(qK)+LHG*sin(qK)-LBC*cos(qB-qK)-LCD*cos(qB-qK)-LDE*cos(qB-qD-qK)-LEF*cos(qB-qD-qK))+sin(qG-qK)*(LHG*cos(qK)-LBH*sin(qK)-LBC*sin(qB-qK)-LCD*sin(qB-qK)-LDE*sin(qB-qD-qK)-LEF*sin(qB-qD-qK)))))-(LBC*sin(qB-qK)+LCI*cos(qB-qK))*((LDE+LEF)*sin(qo2)*cos(qB-qD-qG)*(LKB*cos(qK)+LBC*cos(qB-qK)-LCI*sin(qB-qK))+sin(qo1)*((LDE+LEF)*sin(qo1+qo2)*cos(qB-qD-qG)*(LCI*cos(qB-qK)-LCD*sin(qB-qK)-LDE*sin(qB-qD-qK)-LEJ*cos(qB-qD-qK))-sin(qo1+qo2)*(LDE*sin(qB-qD-qK)+LEJ*cos(qB-qD-qK))*(cos(qG-qK)*(LBH*cos(qK)+LHG*sin(qK)-LBC*cos(qB-qK)-LCD*cos(qB-qK)-LDE*cos(qB-qD-qK)-LEF*cos(qB-qD-qK))+sin(qG-qK)*(LHG*cos(qK)-LBH*sin(qK)-LBC*sin(qB-qK)-LCD*sin(qB-qK)-LDE*sin(qB-qD-qK)-LEF*sin(qB-qD-qK)))-cos(qo1+qo2)*((LDE+LEF)*cos(qG-qK)*cos(qB-qD-qK)*(LCD*cos(qB-qK)+LCI*sin(qB-qK)+LDE*cos(qB-qD-qK)-LEJ*sin(qB-qD-qK))+cos(qG-qK)*(LDE*cos(qB-qD-qK)-LEJ*sin(qB-qD-qK))*(LBH*cos(qK)+LHG*sin(qK)-LBC*cos(qB-qK)-LCD*cos(qB-qK)-LDE*cos(qB-qD-qK)-LEF*cos(qB-qD-qK))+sin(qG-qK)*((LDE+LEF)*sin(qB-qD-qK)*(LCD*cos(qB-qK)+LCI*sin(qB-qK)+LDE*cos(qB-qD-qK)-LEJ*sin(qB-qD-qK))+(LDE*cos(qB-qD-qK)-LEJ*sin(qB-qD-qK))*(LHG*cos(qK)-LBH*sin(qK)-LBC*sin(qB-qK)-LCD*sin(qB-qK)-LDE*sin(qB-qD-qK)-LEF*sin(qB-qD-qK)))))))/(c2*((LDE+LEF)*sin(qo1)*sin(qo2)*cos(qB-qD-qG)*(LIIp*cos(qo1)-c1*sin(qo1))*(LKB*sin(qK)-LBC*sin(qB-qK)-LCI*cos(qB-qK))-cos(qo1)*((LIIp*sin(qo1)+c1*cos(qo1))*((LDE+LEF)*sin(qo2)*cos(qB-qD-qG)*(LKB*sin(qK)-LBC*sin(qB-qK)-LCI*cos(qB-qK))-cos(qo1)*((LDE+LEF)*cos(qB-qD-qG)*(cos(qo1+qo2)*(LCD*cos(qB-qK)+LCI*sin(qB-qK)+LDE*cos(qB-qD-qK)-LEJ*sin(qB-qD-qK))-sin(qo1+qo2)*(LCI*cos(qB-qK)-LCD*sin(qB-qK)-LDE*sin(qB-qD-qK)-LEJ*cos(qB-qD-qK)))+(sin(qo1+qo2)*(LDE*sin(qB-qD-qK)+LEJ*cos(qB-qD-qK))+cos(qo1+qo2)*(LDE*cos(qB-qD-qK)-LEJ*sin(qB-qD-qK)))*(cos(qG-qK)*(LBH*cos(qK)+LHG*sin(qK)-LBC*cos(qB-qK)-LCD*cos(qB-qK)-LDE*cos(qB-qD-qK)-LEF*cos(qB-qD-qK))+sin(qG-qK)*(LHG*cos(qK)-LBH*sin(qK)-LBC*sin(qB-qK)-LCD*sin(qB-qK)-LDE*sin(qB-qD-qK)-LEF*sin(qB-qD-qK)))))-sin(qo1)*(LIIp*cos(qo1)-c1*sin(qo1))*((LDE+LEF)*sin(qo1+qo2)*cos(qB-qD-qG)*(LCI*cos(qB-qK)-LCD*sin(qB-qK)-LDE*sin(qB-qD-qK)-LEJ*cos(qB-qD-qK))-sin(qo1+qo2)*(LDE*sin(qB-qD-qK)+LEJ*cos(qB-qD-qK))*(cos(qG-qK)*(LBH*cos(qK)+LHG*sin(qK)-LBC*cos(qB-qK)-LCD*cos(qB-qK)-LDE*cos(qB-qD-qK)-LEF*cos(qB-qD-qK))+sin(qG-qK)*(LHG*cos(qK)-LBH*sin(qK)-LBC*sin(qB-qK)-LCD*sin(qB-qK)-LDE*sin(qB-qD-qK)-LEF*sin(qB-qD-qK)))-cos(qo1+qo2)*((LDE+LEF)*cos(qG-qK)*cos(qB-qD-qK)*(LCD*cos(qB-qK)+LCI*sin(qB-qK)+LDE*cos(qB-qD-qK)-LEJ*sin(qB-qD-qK))+cos(qG-qK)*(LDE*cos(qB-qD-qK)-LEJ*sin(qB-qD-qK))*(LBH*cos(qK)+LHG*sin(qK)-LBC*cos(qB-qK)-LCD*cos(qB-qK)-LDE*cos(qB-qD-qK)-LEF*cos(qB-qD-qK))+sin(qG-qK)*((LDE+LEF)*sin(qB-qD-qK)*(LCD*cos(qB-qK)+LCI*sin(qB-qK)+LDE*cos(qB-qD-qK)-LEJ*sin(qB-qD-qK))+(LDE*cos(qB-qD-qK)-LEJ*sin(qB-qD-qK))*(LHG*cos(qK)-LBH*sin(qK)-LBC*sin(qB-qK)-LCD*sin(qB-qK)-LDE*sin(qB-qD-qK)-LEF*sin(qB-qD-qK)))))))) - 2*q_dif1*abs(((LDE+LEF)*sin(qo2)*cos(qB-qD-qG)*(LKB*sin(qK)-LBC*sin(qB-qK)-LCI*cos(qB-qK))-cos(qo1)*((LDE+LEF)*cos(qB-qD-qG)*(cos(qo1+qo2)*(LCD*cos(qB-qK)+LCI*sin(qB-qK)+LDE*cos(qB-qD-qK)-LEJ*sin(qB-qD-qK))-sin(qo1+qo2)*(LCI*cos(qB-qK)-LCD*sin(qB-qK)-LDE*sin(qB-qD-qK)-LEJ*cos(qB-qD-qK)))+(sin(qo1+qo2)*(LDE*sin(qB-qD-qK)+LEJ*cos(qB-qD-qK))+cos(qo1+qo2)*(LDE*cos(qB-qD-qK)-LEJ*sin(qB-qD-qK)))*(cos(qG-qK)*(LBH*cos(qK)+LHG*sin(qK)-LBC*cos(qB-qK)-LCD*cos(qB-qK)-LDE*cos(qB-qD-qK)-LEF*cos(qB-qD-qK))+sin(qG-qK)*(LHG*cos(qK)-LBH*sin(qK)-LBC*sin(qB-qK)-LCD*sin(qB-qK)-LDE*sin(qB-qD-qK)-LEF*sin(qB-qD-qK)))))^2*(cos(qN)+sin(qN)^2*((LDE+LEF)*cos(qo1)*sin(qo1+qo2)*cos(qB-qD-qG)*(LKB*sin(qK)-LBC*sin(qB-qK)-LCD*sin(qB-qK)-LDE*sin(qB-qD-qK)-LEJ*cos(qB-qD-qK))-(LDE+LEF)*sin(qo1)*cos(qo1+qo2)*cos(qB-qD-qG)*(LKB*sin(qK)-LBC*sin(qB-qK)-LCI*cos(qB-qK))-cos(qo1)*sin(qo1+qo2)*(LDE*sin(qB-qD-qK)+LEJ*cos(qB-qD-qK))*(cos(qG-qK)*(LBH*cos(qK)+LHG*sin(qK)-LBC*cos(qB-qK)-LCD*cos(qB-qK)-LDE*cos(qB-qD-qK)-LEF*cos(qB-qD-qK))+sin(qG-qK)*(LHG*cos(qK)-LBH*sin(qK)-LBC*sin(qB-qK)-LCD*sin(qB-qK)-LDE*sin(qB-qD-qK)-LEF*sin(qB-qD-qK)))-cos(qo1)*cos(qo1+qo2)*((LDE+LEF)*cos(qG-qK)*cos(qB-qD-qK)*(LCD*cos(qB-qK)+LCI*sin(qB-qK)+LDE*cos(qB-qD-qK)-LEJ*sin(qB-qD-qK))+cos(qG-qK)*(LDE*cos(qB-qD-qK)-LEJ*sin(qB-qD-qK))*(LBH*cos(qK)+LHG*sin(qK)-LBC*cos(qB-qK)-LCD*cos(qB-qK)-LDE*cos(qB-qD-qK)-LEF*cos(qB-qD-qK))+sin(qG-qK)*((LDE+LEF)*sin(qB-qD-qK)*(LCD*cos(qB-qK)+LCI*sin(qB-qK)+LDE*cos(qB-qD-qK)-LEJ*sin(qB-qD-qK))+(LDE*cos(qB-qD-qK)-LEJ*sin(qB-qD-qK))*(LHG*cos(qK)-LBH*sin(qK)-LBC*sin(qB-qK)-LCD*sin(qB-qK)-LDE*sin(qB-qD-qK)-LEF*sin(qB-qD-qK)))))/(cos(qN)*((LDE+LEF)*sin(qo2)*cos(qB-qD-qG)*(LKB*sin(qK)-LBC*sin(qB-qK)-LCI*cos(qB-qK))-cos(qo1)*((LDE+LEF)*cos(qB-qD-qG)*(cos(qo1+qo2)*(LCD*cos(qB-qK)+LCI*sin(qB-qK)+LDE*cos(qB-qD-qK)-LEJ*sin(qB-qD-qK))-sin(qo1+qo2)*(LCI*cos(qB-qK)-LCD*sin(qB-qK)-LDE*sin(qB-qD-qK)-LEJ*cos(qB-qD-qK)))+(sin(qo1+qo2)*(LDE*sin(qB-qD-qK)+LEJ*cos(qB-qD-qK))+cos(qo1+qo2)*(LDE*cos(qB-qD-qK)-LEJ*sin(qB-qD-qK)))*(cos(qG-qK)*(LBH*cos(qK)+LHG*sin(qK)-LBC*cos(qB-qK)-LCD*cos(qB-qK)-LDE*cos(qB-qD-qK)-LEF*cos(qB-qD-qK))+sin(qG-qK)*(LHG*cos(qK)-LBH*sin(qK)-LBC*sin(qB-qK)-LCD*sin(qB-qK)-LDE*sin(qB-qD-qK)-LEF*sin(qB-qD-qK)))))))*(LIIp*sin(qo1)+c1*cos(qo1)+((LDE+LEF)*c2*cos(qB-qD-qG)*(cos(qo1)*(LKB*cos(qK)+LBC*cos(qB-qK)-LCI*sin(qB-qK))-sin(qo1)*(LKB*sin(qK)-LBC*sin(qB-qK)-LCI*cos(qB-qK)))+(LDE+LEF)*sin(qo1+qo2)*cos(qB-qD-qG)*(LIIp*cos(qo1)+sin(qo1)*(LLM-c1))*(cos(qo1)*(LKB*cos(qK)+LBC*cos(qB-qK)-LCI*sin(qB-qK))-sin(qo1)*(LKB*sin(qK)-LBC*sin(qB-qK)-LCI*cos(qB-qK)))-(LDE+LEF)*cos(qo1+qo2)*cos(qB-qD-qG)*(LIIp*sin(qo1)-cos(qo1)*(LLM-c1))*(cos(qo1)*(LKB*cos(qK)+LBC*cos(qB-qK)-LCI*sin(qB-qK))-sin(qo1)*(LKB*sin(qK)-LBC*sin(qB-qK)-LCI*cos(qB-qK)))-(LIIp*cos(qo1)-c1*sin(qo1))*((LDE+LEF)*sin(qo2)*cos(qB-qD-qG)*(LKB*cos(qK)+LBC*cos(qB-qK)-LCI*sin(qB-qK))+sin(qo1)*((LDE+LEF)*sin(qo1+qo2)*cos(qB-qD-qG)*(LCI*cos(qB-qK)-LCD*sin(qB-qK)-LDE*sin(qB-qD-qK)-LEJ*cos(qB-qD-qK))-sin(qo1+qo2)*(LDE*sin(qB-qD-qK)+LEJ*cos(qB-qD-qK))*(cos(qG-qK)*(LBH*cos(qK)+LHG*sin(qK)-LBC*cos(qB-qK)-LCD*cos(qB-qK)-LDE*cos(qB-qD-qK)-LEF*cos(qB-qD-qK))+sin(qG-qK)*(LHG*cos(qK)-LBH*sin(qK)-LBC*sin(qB-qK)-LCD*sin(qB-qK)-LDE*sin(qB-qD-qK)-LEF*sin(qB-qD-qK)))-cos(qo1+qo2)*((LDE+LEF)*cos(qG-qK)*cos(qB-qD-qK)*(LCD*cos(qB-qK)+LCI*sin(qB-qK)+LDE*cos(qB-qD-qK)-LEJ*sin(qB-qD-qK))+cos(qG-qK)*(LDE*cos(qB-qD-qK)-LEJ*sin(qB-qD-qK))*(LBH*cos(qK)+LHG*sin(qK)-LBC*cos(qB-qK)-LCD*cos(qB-qK)-LDE*cos(qB-qD-qK)-LEF*cos(qB-qD-qK))+sin(qG-qK)*((LDE+LEF)*sin(qB-qD-qK)*(LCD*cos(qB-qK)+LCI*sin(qB-qK)+LDE*cos(qB-qD-qK)-LEJ*sin(qB-qD-qK))+(LDE*cos(qB-qD-qK)-LEJ*sin(qB-qD-qK))*(LHG*cos(qK)-LBH*sin(qK)-LBC*sin(qB-qK)-LCD*sin(qB-qK)-LDE*sin(qB-qD-qK)-LEF*sin(qB-qD-qK)))))))/((LDE+LEF)*sin(qo2)*cos(qB-qD-qG)*(LKB*sin(qK)-LBC*sin(qB-qK)-LCI*cos(qB-qK))-cos(qo1)*((LDE+LEF)*cos(qB-qD-qG)*(cos(qo1+qo2)*(LCD*cos(qB-qK)+LCI*sin(qB-qK)+LDE*cos(qB-qD-qK)-LEJ*sin(qB-qD-qK))-sin(qo1+qo2)*(LCI*cos(qB-qK)-LCD*sin(qB-qK)-LDE*sin(qB-qD-qK)-LEJ*cos(qB-qD-qK)))+(sin(qo1+qo2)*(LDE*sin(qB-qD-qK)+LEJ*cos(qB-qD-qK))+cos(qo1+qo2)*(LDE*cos(qB-qD-qK)-LEJ*sin(qB-qD-qK)))*(cos(qG-qK)*(LBH*cos(qK)+LHG*sin(qK)-LBC*cos(qB-qK)-LCD*cos(qB-qK)-LDE*cos(qB-qD-qK)-LEF*cos(qB-qD-qK))+sin(qG-qK)*(LHG*cos(qK)-LBH*sin(qK)-LBC*sin(qB-qK)-LCD*sin(qB-qK)-LDE*sin(qB-qD-qK)-LEF*sin(qB-qD-qK))))))/((LDE+LEF)*c2*cos(qB-qD-qG)*(LKB*sin(qK)+LAB*sin(qB-qK)-tan(qN)*(LKB*cos(qK)-LAB*cos(qB-qK)))*((LDE+LEF)*sin(qo1)*sin(qo2)*cos(qB-qD-qG)*(LIIp*cos(qo1)-c1*sin(qo1))*(LKB*sin(qK)-LBC*sin(qB-qK)-LCI*cos(qB-qK))-cos(qo1)*((LIIp*sin(qo1)+c1*cos(qo1))*((LDE+LEF)*sin(qo2)*cos(qB-qD-qG)*(LKB*sin(qK)-LBC*sin(qB-qK)-LCI*cos(qB-qK))-cos(qo1)*((LDE+LEF)*cos(qB-qD-qG)*(cos(qo1+qo2)*(LCD*cos(qB-qK)+LCI*sin(qB-qK)+LDE*cos(qB-qD-qK)-LEJ*sin(qB-qD-qK))-sin(qo1+qo2)*(LCI*cos(qB-qK)-LCD*sin(qB-qK)-LDE*sin(qB-qD-qK)-LEJ*cos(qB-qD-qK)))+(sin(qo1+qo2)*(LDE*sin(qB-qD-qK)+LEJ*cos(qB-qD-qK))+cos(qo1+qo2)*(LDE*cos(qB-qD-qK)-LEJ*sin(qB-qD-qK)))*(cos(qG-qK)*(LBH*cos(qK)+LHG*sin(qK)-LBC*cos(qB-qK)-LCD*cos(qB-qK)-LDE*cos(qB-qD-qK)-LEF*cos(qB-qD-qK))+sin(qG-qK)*(LHG*cos(qK)-LBH*sin(qK)-LBC*sin(qB-qK)-LCD*sin(qB-qK)-LDE*sin(qB-qD-qK)-LEF*sin(qB-qD-qK)))))-sin(qo1)*(LIIp*cos(qo1)-c1*sin(qo1))*((LDE+LEF)*sin(qo1+qo2)*cos(qB-qD-qG)*(LCI*cos(qB-qK)-LCD*sin(qB-qK)-LDE*sin(qB-qD-qK)-LEJ*cos(qB-qD-qK))-sin(qo1+qo2)*(LDE*sin(qB-qD-qK)+LEJ*cos(qB-qD-qK))*(cos(qG-qK)*(LBH*cos(qK)+LHG*sin(qK)-LBC*cos(qB-qK)-LCD*cos(qB-qK)-LDE*cos(qB-qD-qK)-LEF*cos(qB-qD-qK))+sin(qG-qK)*(LHG*cos(qK)-LBH*sin(qK)-LBC*sin(qB-qK)-LCD*sin(qB-qK)-LDE*sin(qB-qD-qK)-LEF*sin(qB-qD-qK)))-cos(qo1+qo2)*((LDE+LEF)*cos(qG-qK)*cos(qB-qD-qK)*(LCD*cos(qB-qK)+LCI*sin(qB-qK)+LDE*cos(qB-qD-qK)-LEJ*sin(qB-qD-qK))+cos(qG-qK)*(LDE*cos(qB-qD-qK)-LEJ*sin(qB-qD-qK))*(LBH*cos(qK)+LHG*sin(qK)-LBC*cos(qB-qK)-LCD*cos(qB-qK)-LDE*cos(qB-qD-qK)-LEF*cos(qB-qD-qK))+sin(qG-qK)*((LDE+LEF)*sin(qB-qD-qK)*(LCD*cos(qB-qK)+LCI*sin(qB-qK)+LDE*cos(qB-qD-qK)-LEJ*sin(qB-qD-qK))+(LDE*cos(qB-qD-qK)-LEJ*sin(qB-qD-qK))*(LHG*cos(qK)-LBH*sin(qK)-LBC*sin(qB-qK)-LCD*sin(qB-qK)-LDE*sin(qB-qD-qK)-LEF*sin(qB-qD-qK)))))))))/q_dif2 - ((LDE+LEF)*sin(qo2)*cos(qB-qD-qG)*(LKB*sin(qK)-LBC*sin(qB-qK)-LCI*cos(qB-qK))-cos(qo1)*((LDE+LEF)*cos(qB-qD-qG)*(cos(qo1+qo2)*(LCD*cos(qB-qK)+LCI*sin(qB-qK)+LDE*cos(qB-qD-qK)-LEJ*sin(qB-qD-qK))-sin(qo1+qo2)*(LCI*cos(qB-qK)-LCD*sin(qB-qK)-LDE*sin(qB-qD-qK)-LEJ*cos(qB-qD-qK)))+(sin(qo1+qo2)*(LDE*sin(qB-qD-qK)+LEJ*cos(qB-qD-qK))+cos(qo1+qo2)*(LDE*cos(qB-qD-qK)-LEJ*sin(qB-qD-qK)))*(cos(qG-qK)*(LBH*cos(qK)+LHG*sin(qK)-LBC*cos(qB-qK)-LCD*cos(qB-qK)-LDE*cos(qB-qD-qK)-LEF*cos(qB-qD-qK))+sin(qG-qK)*(LHG*cos(qK)-LBH*sin(qK)-LBC*sin(qB-qK)-LCD*sin(qB-qK)-LDE*sin(qB-qD-qK)-LEF*sin(qB-qD-qK)))))^2*(LIIp*sin(qo1)+c1*cos(qo1)+((LDE+LEF)*c2*cos(qB-qD-qG)*(cos(qo1)*(LKB*cos(qK)+LBC*cos(qB-qK)-LCI*sin(qB-qK))-sin(qo1)*(LKB*sin(qK)-LBC*sin(qB-qK)-LCI*cos(qB-qK)))+(LDE+LEF)*sin(qo1+qo2)*cos(qB-qD-qG)*(LIIp*cos(qo1)+sin(qo1)*(LLM-c1))*(cos(qo1)*(LKB*cos(qK)+LBC*cos(qB-qK)-LCI*sin(qB-qK))-sin(qo1)*(LKB*sin(qK)-LBC*sin(qB-qK)-LCI*cos(qB-qK)))-(LDE+LEF)*cos(qo1+qo2)*cos(qB-qD-qG)*(LIIp*sin(qo1)-cos(qo1)*(LLM-c1))*(cos(qo1)*(LKB*cos(qK)+LBC*cos(qB-qK)-LCI*sin(qB-qK))-sin(qo1)*(LKB*sin(qK)-LBC*sin(qB-qK)-LCI*cos(qB-qK)))-(LIIp*cos(qo1)-c1*sin(qo1))*((LDE+LEF)*sin(qo2)*cos(qB-qD-qG)*(LKB*cos(qK)+LBC*cos(qB-qK)-LCI*sin(qB-qK))+sin(qo1)*((LDE+LEF)*sin(qo1+qo2)*cos(qB-qD-qG)*(LCI*cos(qB-qK)-LCD*sin(qB-qK)-LDE*sin(qB-qD-qK)-LEJ*cos(qB-qD-qK))-sin(qo1+qo2)*(LDE*sin(qB-qD-qK)+LEJ*cos(qB-qD-qK))*(cos(qG-qK)*(LBH*cos(qK)+LHG*sin(qK)-LBC*cos(qB-qK)-LCD*cos(qB-qK)-LDE*cos(qB-qD-qK)-LEF*cos(qB-qD-qK))+sin(qG-qK)*(LHG*cos(qK)-LBH*sin(qK)-LBC*sin(qB-qK)-LCD*sin(qB-qK)-LDE*sin(qB-qD-qK)-LEF*sin(qB-qD-qK)))-cos(qo1+qo2)*((LDE+LEF)*cos(qG-qK)*cos(qB-qD-qK)*(LCD*cos(qB-qK)+LCI*sin(qB-qK)+LDE*cos(qB-qD-qK)-LEJ*sin(qB-qD-qK))+cos(qG-qK)*(LDE*cos(qB-qD-qK)-LEJ*sin(qB-qD-qK))*(LBH*cos(qK)+LHG*sin(qK)-LBC*cos(qB-qK)-LCD*cos(qB-qK)-LDE*cos(qB-qD-qK)-LEF*cos(qB-qD-qK))+sin(qG-qK)*((LDE+LEF)*sin(qB-qD-qK)*(LCD*cos(qB-qK)+LCI*sin(qB-qK)+LDE*cos(qB-qD-qK)-LEJ*sin(qB-qD-qK))+(LDE*cos(qB-qD-qK)-LEJ*sin(qB-qD-qK))*(LHG*cos(qK)-LBH*sin(qK)-LBC*sin(qB-qK)-LCD*sin(qB-qK)-LDE*sin(qB-qD-qK)-LEF*sin(qB-qD-qK)))))))/((LDE+LEF)*sin(qo2)*cos(qB-qD-qG)*(LKB*sin(qK)-LBC*sin(qB-qK)-LCI*cos(qB-qK))-cos(qo1)*((LDE+LEF)*cos(qB-qD-qG)*(cos(qo1+qo2)*(LCD*cos(qB-qK)+LCI*sin(qB-qK)+LDE*cos(qB-qD-qK)-LEJ*sin(qB-qD-qK))-sin(qo1+qo2)*(LCI*cos(qB-qK)-LCD*sin(qB-qK)-LDE*sin(qB-qD-qK)-LEJ*cos(qB-qD-qK)))+(sin(qo1+qo2)*(LDE*sin(qB-qD-qK)+LEJ*cos(qB-qD-qK))+cos(qo1+qo2)*(LDE*cos(qB-qD-qK)-LEJ*sin(qB-qD-qK)))*(cos(qG-qK)*(LBH*cos(qK)+LHG*sin(qK)-LBC*cos(qB-qK)-LCD*cos(qB-qK)-LDE*cos(qB-qD-qK)-LEF*cos(qB-qD-qK))+sin(qG-qK)*(LHG*cos(qK)-LBH*sin(qK)-LBC*sin(qB-qK)-LCD*sin(qB-qK)-LDE*sin(qB-qD-qK)-LEF*sin(qB-qD-qK))))))*(LAB*sin(qB-qK)-((LDE+LEF)*cos(qo1)*sin(qo1+qo2)*cos(qB-qD-qG)*(LKB*sin(qK)+LAB*sin(qB-qK)-tan(qN)*(LKB*cos(qK)-LAB*cos(qB-qK)))*(LCI*cos(qB-qK)-LCD*sin(qB-qK)-LDE*sin(qB-qD-qK)-LEJ*cos(qB-qD-qK))+cos(qo1)*sin(qG-qK)*(LKB*sin(qK)+LAB*sin(qB-qK)-tan(qN)*(LKB*cos(qK)-LAB*cos(qB-qK)))*(LBC*sin(qB-qK)+LCD*sin(qB-qK)+LDE*sin(qB-qD-qK)+LEF*sin(qB-qD-qK))*(sin(qo1+qo2)*(LDE*sin(qB-qD-qK)+LEJ*cos(qB-qD-qK))+cos(qo1+qo2)*(LDE*cos(qB-qD-qK)-LEJ*sin(qB-qD-qK)))+cos(qo1)*cos(qG-qK)*(LKB*sin(qK)+LAB*sin(qB-qK)-tan(qN)*(LKB*cos(qK)-LAB*cos(qB-qK)))*(LBC*cos(qB-qK)+LCD*cos(qB-qK)+LDE*cos(qB-qD-qK)+LEF*cos(qB-qD-qK))*(sin(qo1+qo2)*(LDE*sin(qB-qD-qK)+LEJ*cos(qB-qD-qK))+cos(qo1+qo2)*(LDE*cos(qB-qD-qK)-LEJ*sin(qB-qD-qK)))-(LDE+LEF)*sin(qo2)*cos(qB-qD-qG)*(LBC*sin(qB-qK)+LCI*cos(qB-qK))*(LKB*sin(qK)+LAB*sin(qB-qK)-tan(qN)*(LKB*cos(qK)-LAB*cos(qB-qK)))-(LDE+LEF)*cos(qo1)*cos(qo1+qo2)*cos(qB-qD-qG)*(LKB*sin(qK)+LAB*sin(qB-qK)-tan(qN)*(LKB*cos(qK)-LAB*cos(qB-qK)))*(LCD*cos(qB-qK)+LCI*sin(qB-qK)+LDE*cos(qB-qD-qK)-LEJ*sin(qB-qD-qK))-LAB*tan(qN)*cos(qB-qK)*((LDE+LEF)*cos(qo1)*sin(qo1+qo2)*cos(qB-qD-qG)*(LKB*sin(qK)-LBC*sin(qB-qK)-LCD*sin(qB-qK)-LDE*sin(qB-qD-qK)-LEJ*cos(qB-qD-qK))-(LDE+LEF)*sin(qo1)*cos(qo1+qo2)*cos(qB-qD-qG)*(LKB*sin(qK)-LBC*sin(qB-qK)-LCI*cos(qB-qK))-cos(qo1)*sin(qo1+qo2)*(LDE*sin(qB-qD-qK)+LEJ*cos(qB-qD-qK))*(cos(qG-qK)*(LBH*cos(qK)+LHG*sin(qK)-LBC*cos(qB-qK)-LCD*cos(qB-qK)-LDE*cos(qB-qD-qK)-LEF*cos(qB-qD-qK))+sin(qG-qK)*(LHG*cos(qK)-LBH*sin(qK)-LBC*sin(qB-qK)-LCD*sin(qB-qK)-LDE*sin(qB-qD-qK)-LEF*sin(qB-qD-qK)))-cos(qo1)*cos(qo1+qo2)*((LDE+LEF)*cos(qG-qK)*cos(qB-qD-qK)*(LCD*cos(qB-qK)+LCI*sin(qB-qK)+LDE*cos(qB-qD-qK)-LEJ*sin(qB-qD-qK))+cos(qG-qK)*(LDE*cos(qB-qD-qK)-LEJ*sin(qB-qD-qK))*(LBH*cos(qK)+LHG*sin(qK)-LBC*cos(qB-qK)-LCD*cos(qB-qK)-LDE*cos(qB-qD-qK)-LEF*cos(qB-qD-qK))+sin(qG-qK)*((LDE+LEF)*sin(qB-qD-qK)*(LCD*cos(qB-qK)+LCI*sin(qB-qK)+LDE*cos(qB-qD-qK)-LEJ*sin(qB-qD-qK))+(LDE*cos(qB-qD-qK)-LEJ*sin(qB-qD-qK))*(LHG*cos(qK)-LBH*sin(qK)-LBC*sin(qB-qK)-LCD*sin(qB-qK)-LDE*sin(qB-qD-qK)-LEF*sin(qB-qD-qK))))))/((LDE+LEF)*sin(qo2)*cos(qB-qD-qG)*(LKB*sin(qK)-LBC*sin(qB-qK)-LCI*cos(qB-qK))-cos(qo1)*((LDE+LEF)*cos(qB-qD-qG)*(cos(qo1+qo2)*(LCD*cos(qB-qK)+LCI*sin(qB-qK)+LDE*cos(qB-qD-qK)-LEJ*sin(qB-qD-qK))-sin(qo1+qo2)*(LCI*cos(qB-qK)-LCD*sin(qB-qK)-LDE*sin(qB-qD-qK)-LEJ*cos(qB-qD-qK)))+(sin(qo1+qo2)*(LDE*sin(qB-qD-qK)+LEJ*cos(qB-qD-qK))+cos(qo1+qo2)*(LDE*cos(qB-qD-qK)-LEJ*sin(qB-qD-qK)))*(cos(qG-qK)*(LBH*cos(qK)+LHG*sin(qK)-LBC*cos(qB-qK)-LCD*cos(qB-qK)-LDE*cos(qB-qD-qK)-LEF*cos(qB-qD-qK))+sin(qG-qK)*(LHG*cos(qK)-LBH*sin(qK)-LBC*sin(qB-qK)-LCD*sin(qB-qK)-LDE*sin(qB-qD-qK)-LEF*sin(qB-qD-qK))))))/((LDE+LEF)*c2*cos(qB-qD-qG)*(LKB*sin(qK)+LAB*sin(qB-qK)-tan(qN)*(LKB*cos(qK)-LAB*cos(qB-qK)))*((LDE+LEF)*sin(qo1)*sin(qo2)*cos(qB-qD-qG)*(LIIp*cos(qo1)-c1*sin(qo1))*(LKB*sin(qK)-LBC*sin(qB-qK)-LCI*cos(qB-qK))-cos(qo1)*((LIIp*sin(qo1)+c1*cos(qo1))*((LDE+LEF)*sin(qo2)*cos(qB-qD-qG)*(LKB*sin(qK)-LBC*sin(qB-qK)-LCI*cos(qB-qK))-cos(qo1)*((LDE+LEF)*cos(qB-qD-qG)*(cos(qo1+qo2)*(LCD*cos(qB-qK)+LCI*sin(qB-qK)+LDE*cos(qB-qD-qK)-LEJ*sin(qB-qD-qK))-sin(qo1+qo2)*(LCI*cos(qB-qK)-LCD*sin(qB-qK)-LDE*sin(qB-qD-qK)-LEJ*cos(qB-qD-qK)))+(sin(qo1+qo2)*(LDE*sin(qB-qD-qK)+LEJ*cos(qB-qD-qK))+cos(qo1+qo2)*(LDE*cos(qB-qD-qK)-LEJ*sin(qB-qD-qK)))*(cos(qG-qK)*(LBH*cos(qK)+LHG*sin(qK)-LBC*cos(qB-qK)-LCD*cos(qB-qK)-LDE*cos(qB-qD-qK)-LEF*cos(qB-qD-qK))+sin(qG-qK)*(LHG*cos(qK)-LBH*sin(qK)-LBC*sin(qB-qK)-LCD*sin(qB-qK)-LDE*sin(qB-qD-qK)-LEF*sin(qB-qD-qK)))))-sin(qo1)*(LIIp*cos(qo1)-c1*sin(qo1))*((LDE+LEF)*sin(qo1+qo2)*cos(qB-qD-qG)*(LCI*cos(qB-qK)-LCD*sin(qB-qK)-LDE*sin(qB-qD-qK)-LEJ*cos(qB-qD-qK))-sin(qo1+qo2)*(LDE*sin(qB-qD-qK)+LEJ*cos(qB-qD-qK))*(cos(qG-qK)*(LBH*cos(qK)+LHG*sin(qK)-LBC*cos(qB-qK)-LCD*cos(qB-qK)-LDE*cos(qB-qD-qK)-LEF*cos(qB-qD-qK))+sin(qG-qK)*(LHG*cos(qK)-LBH*sin(qK)-LBC*sin(qB-qK)-LCD*sin(qB-qK)-LDE*sin(qB-qD-qK)-LEF*sin(qB-qD-qK)))-cos(qo1+qo2)*((LDE+LEF)*cos(qG-qK)*cos(qB-qD-qK)*(LCD*cos(qB-qK)+LCI*sin(qB-qK)+LDE*cos(qB-qD-qK)-LEJ*sin(qB-qD-qK))+cos(qG-qK)*(LDE*cos(qB-qD-qK)-LEJ*sin(qB-qD-qK))*(LBH*cos(qK)+LHG*sin(qK)-LBC*cos(qB-qK)-LCD*cos(qB-qK)-LDE*cos(qB-qD-qK)-LEF*cos(qB-qD-qK))+sin(qG-qK)*((LDE+LEF)*sin(qB-qD-qK)*(LCD*cos(qB-qK)+LCI*sin(qB-qK)+LDE*cos(qB-qD-qK)-LEJ*sin(qB-qD-qK))+(LDE*cos(qB-qD-qK)-LEJ*sin(qB-qD-qK))*(LHG*cos(qK)-LBH*sin(qK)-LBC*sin(qB-qK)-LCD*sin(qB-qK)-LDE*sin(qB-qD-qK)-LEF*sin(qB-qD-qK)))))))))/2;

if J22_c == 0 || isnan(J22_c) || isinf(J22_c)
    J22 = single(J22_old);
else
    J22 = single(J22_c); % Non ricordo perch\'e l'avevo scritto così -abs(J22_c));
end
% 
J22_ol = single(J22);



JTcomp = [J11; J12; J21; J22];


q_next = single(sensor);

== matlab function dx_hand_model_rai3/Thumb/Metacarphal Phalanx/MATLAB Function4 ==
  data: u input; d output
function d = fcn(u)

d = sqrt(u(1)^2+u(2)^2+u(3)^2);

== matlab function dx_hand_model_rai3/Middle Finger/Position-Force Architecture/Optimized_Static_Problem ==
  data: Jcomponents input; y output; force_vector input
function y = fcn(Jcomponents, force_vector)
% Utilizzo la rendering strategy in the Force Space proposta da Mine
j_f = [0;0];
j_f = [force_vector(1);force_vector(2)];

Ja = [single(Jcomponents(1)); single(Jcomponents(3))];
Jp = [single(Jcomponents(2)); single(Jcomponents(4))];

% J = [Ja Jp];

a_f = Ja'*(eye(2)-Jp*inv(Jp'*Jp)*Jp')*j_f;

y = a_f;

== matlab function dx_hand_model_rai3/Middle Finger/Pose Generator/Middle Direct Kinematics ==
  data: u input; y output; measurements input
function y  = fcn(u, measurements)
%#codegen


% vecchi
% LKN =  135.6320;
% qKN = 0.1108;
% lact = 117.77;
s_slitta = 13.5; % [mm] misurato con il calibro

xL_mag = measurements(3); % Posizione lungo l'asse x di L rispetto a K [RIMISURA]
offset = measurements(4); % Distanza tra il giunto K e l'appoggio del metacarpo [RIMISURA]
LIIp = measurements(1); % Semispessore del metacarpo e della falange (da tarare)
LJJp = LIIp; % semispessore della falangina (da tarare, non per forza uguale a LIIp)
LLM = measurements(2); % Lunghezza della falange
LAB =  measurements(5);
LBC =  measurements(6);
LCD =  measurements(7);
LDE =  measurements(8);
LEF =  measurements(9);
LBH =  measurements(10); 
LGH =  measurements(11);
LGF =  measurements(12);
LEJ =  measurements(13);
LCI =  measurements(14);
LKB =  measurements(15);
LKNy = measurements(16); %% MISURA
LKNx = measurements(17); %% MISURA
lact = measurements(18); %Lunghezza dell'attuatore. [RIMISURA]

LKH = LKB + LBH;
LDF = LDE + LEF;
LBD = LBC + LCD;

LKN =  sqrt(LKNx^2 + LKNy^2); %135.6320;
qKN = atan(LKNy / LKNx); %0.1108; % angolo tra il giunto dell'attacco del motore (N) e il giunto K 



xL = -xL_mag; % Derivata  
yL = -(offset); % Distanza tra K e 01

lx = u(1); % Allungamento del motore misurato
qB = u(2); % Angolo inB misurato dal potenziometro (espresso in radianti)

LAK = sqrt(LAB^2 + LKB^2 - 2*LAB*LKB*cos(qB)); % quadrato della distanza tra A e K. Non può venire mai negativo

%% Calcolo qK
% Calcolo di qN: l'angolo del motore (mia implementazione). Non può mai
% essere negarivo
qN = my_acos( (- LAK^2 + LKN^2 + (lx+lact)^2)/(2*(lx+lact)*LKN) ) ;

% Coseno dell'angolo in K del triangolo AKB
xK1 = (-LAB^2 + LAK^2 + LKB^2)/(2*LAK*LKB); 
qK1 = my_acos(xK1);

% Coseno dell'angolo in K del triangolo AKN
xK2 = (-(lx+lact)^2 + LAK^2 + LKN^2)/(2*LAK*LKN);
qK2 = my_acos(xK2);

% Angolo qK
qK = pi - ( qK1 + qK2 + qKN);

%% Calcolo coordinate punti cinematica parallela
% il centro del sistema di riferimento è in K con asse x verso il polso e
% asse y uscente (contratio alle dita)

% punto B
xB = - LKB * cos(qK);  yB = LKB * sin(qK);
% punto H
xH = - LKH * cos(qK);  yH = LKH * sin(qK);
% punto G
xG = xH - LGH*sin(qK);  yG = yH - LGH*cos(qK);
% punto C
xC = xB - LBC*cos(qB - qK); yC = yB - LBC * sin(qB - qK);
% punto D
xD = xC - LCD*cos(qB - qK);   yD = yC - LCD*sin(qB - qK);
% punto I
xI = xC + LCI * sin(qB - qK);   yI = yC - LCI * cos(qB - qK);
% distanza tra L ed I
LLI = sqrt((xI - xL)^2 + (yI - yL)^2);


%% C1: dello slider. Distanza I da L proiettato sullo slider
spessore = LIIp + s_slitta;
temp = LLI^2 - spessore^2;

if (temp < 0)
    temp = single(0);
end
c1 = sqrt(temp);

% angolo in L del triangolo LIU
xj1 = (-spessore^2 + LLI^2 + c1^2)/(2*c1*LLI);
if abs(xj1)>1
    xj1 = single(1);
end
qj1 = abs(my_acos(xj1));

%% calcolo di qo1

alpha = atan((yL - yI)/(xL - xI));
qo1 = qj1 + alpha;
    
%% Calcolo distanze tra punti nella cinematica parallela   
LHD = sqrt((xH - xD)^2 + (yH - yD)^2);
LDG = sqrt((xG - xD)^2 + (yG - yD)^2);


% angolo in G triangolo DGH - puo' diventare ottuso
xG1 = (-LHD^2 + LDG^2 + LGH^2)/(2*LDG*LGH);
if abs(xG1)>1
    xG1=single(1);
end
qG1 = abs(my_acos(xG1));
% angolo in G triangolo FGD - non puo' diventare ottuso
xG2 = (-LDF^2 + LDG^2 + LGF^2)/(2*LDG*LGF);
if abs(xG2)>1
    xG2=single(1);
end

qG2 = abs(my_acos(xG2));
qG = pi - (qG1 + qG2);

%% Seconda falange
% Giunto M del dito
xM = xL - LLM*cos(qo1); yM = yL - LLM*sin(qo1);

% Angolo in D triangolo DGH
xD1 = (-LGH^2 + LHD^2 + LDG^2)/(2*LHD*LDG);
if abs(xD1)>1
    xD1=single(1);
end
qD1 = abs(my_acos(xD1));
% Angolo in D triangolo GFD
xD2 = (-LGF^2 + LDG^2 + LDF^2)/(2*LDG*LDF);
if abs(xD2)>1
    xD2=single(1);
end
qD2 = abs(my_acos(xD2));
% Angolo in D triangolo BDH
xD3 = (-LBH^2 + LHD^2 + LBD^2)/(2*LHD*LBD);
if abs(xD3)>1
    xD3=single(1);
end
qD3 = abs(my_acos(xD3));

qD = pi - (qD1 + qD2 + qD3);

% Giunto E
xE = xD - LDE*cos(qB - qD - qK);
yE = yD - LDE*sin(qB - qD - qK);
% Giunto J
xJ = xE + LEJ*sin(qB - qD - qK);  
yJ = yE - LEJ*cos(qB - qD - qK);
% Distanza JM
LJM = sqrt((xJ - xM)^2 + (yJ - yM)^2);
% calcolo c2
temp = LJM^2 - spessore^2;
if temp < 0
    temp = single(0);
end
c2 = sqrt(temp);

% Angolo in M triangolo JSM
xj2 = (-spessore^2 + LJM^2 + c2^2)/(2*c2*LJM);
if abs(xj2)>1
    xj2=single(1);
end
qj2 = abs(my_acos(xj2));


% if (xJ - xM)<=0
    qj3 = atan2((yM - yJ),(xM - xJ));
% else
%     qj3 = pi + atan((yJ - yM)/(xJ - xM));
% end


qo2 = qj2 + qj3 - qo1;

LIJ = sqrt((xI-xJ)^2 + (yI-yJ)^2);
LBJ = sqrt((xB-xJ)^2 + (yB-yJ)^2);


y = [qo1; qo2; qK; qD; qG; qN; c1; c2];

% y = [qo1; qo2; qK; qD; xI; xL; yI; yL;LLI];
end
%% my_acos
function y = my_acos(x)
%     if x < 1
%         t = single(1);
%     else
%         if x > 1
%             t = single(1);
%         else
%             t = x;
%         end
%     end
%   
    t = complex(x);
    y = real( acos(t) );
            
end

== matlab function dx_hand_model_rai3/Middle Finger/Position-Force Architecture/Classic_Static_Problem ==
  data: Jcomponents input; y output; force_vector input
function y = fcn(Jcomponents, force_vector)
% Utilizzo la rendering strategy in the Force Space proposta da Mine
j_f = [force_vector(1);force_vector(2)];

Ja = [single(Jcomponents(1)); single(Jcomponents(3))];
% Jp = [single(Jcomponents(2)); single(Jcomponents(4))];

% J = [Ja Jp];

a_f = Ja'*j_f;

y = a_f;
